simulink model "Questao_5"  (R2023b)
settings: Solver=VariableStepAuto  StartTime=0.0  StopTime=100  RelTol=1e-3
undefined symbols (not defined in the file): B, Kw, Ts
settings Model: Creator=pedro  LastModifiedBy=pedro

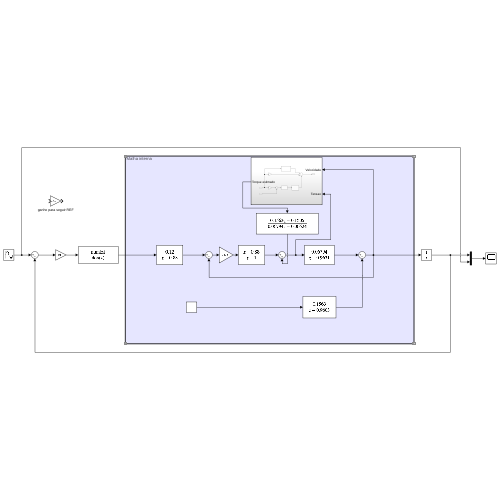
[thumbnail: Simulink's stored preview of the top-level diagram]
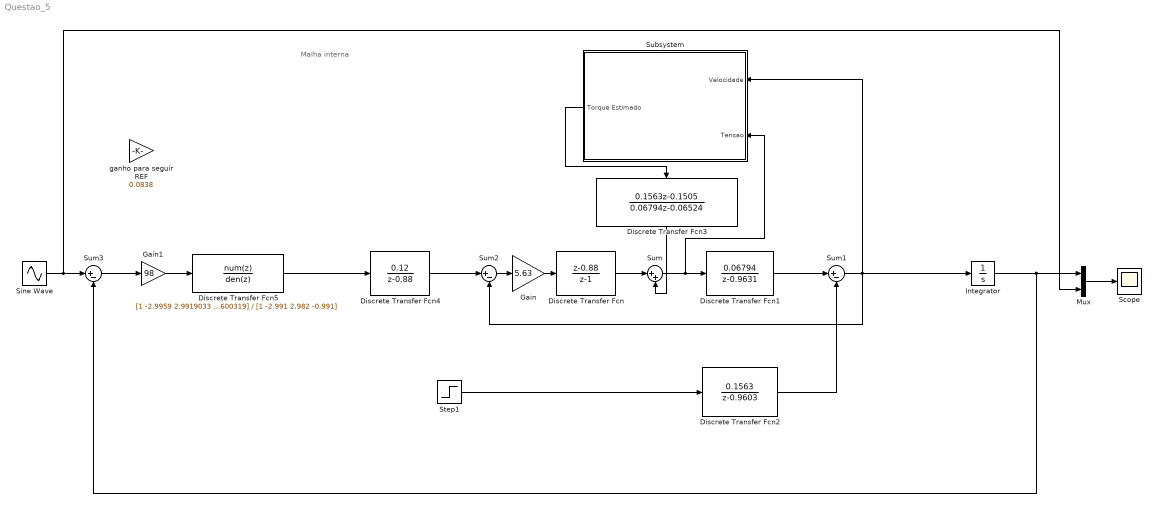
== system Questao_5 ==
  note: Malha interna
  Discrete Transfer Fcn : DiscreteTransferFcn  Numerator=[1 -0.88]  Denominator=[1 -1]
  Discrete Transfer Fcn1 : DiscreteTransferFcn  Numerator=[0.06794]  Denominator=[1 -0.9631]
  Discrete Transfer Fcn2 : DiscreteTransferFcn  Numerator=[0.1563]  Denominator=[1 -0.9603]
  Discrete Transfer Fcn3 : DiscreteTransferFcn  Numerator=[0.1563 -0.1505]  Denominator=[0.06794 -0.06524]
  Discrete Transfer Fcn4 : DiscreteTransferFcn  Numerator=[0.12]  Denominator=[1 -0.88]
  Discrete Transfer Fcn5 : DiscreteTransferFcn  Numerator=[1 -2.9959 2.9919033 -0.99600319]  Denominator=[1 -2.991 2.982 -0.991]
  Gain : Gain  Gain=5.63
  Gain1 : Gain  Gain=98
  Integrator : Integrator
  Mux : Mux  Inputs=2
  Scope : Scope
  Sine Wave : Sin  SampleTime=0.162
  Step1 : Step  Time=10  After=0  SampleTime=0.162
  Subsystem : Subsystem
      settings: PortSchema="{\"entries\":[{\"content\":{\"sides\":[{\"content\":{},\"type\":\"ConnectorPlacement.EquallySpacedRectSide\",\"uuid\":\"e59a06e1-eab4-4bd2-85d9-68e257427de7\"},{\"content\":{\"side\":\"RIGHT\"},\"type\":\"ConnectorPlacement.EquallySpacedRectSide\",\"uuid\":\"6892985a-c8d8-4c3b-9c0c-3e543d6e16eb\"},{\"content\":{\"connectorIds\":[\"Out1\"],\"side\":\"TOP\"},\"type\":\"ConnectorPlacement.EquallySpacedRectSide\",\"uuid\":\"71dba93a-139c-4e39-b2a6-d594bacb8791\"},{\"content\":{\"connectorIds\":[\"In1\",\"In2\"],\"side\":\"BOTTOM\"},\"type\":\"ConnectorPlacement.EquallySpacedRectSide\",\"uuid\":\"1da54c87-6e6c-45c2-97e0-448bf39b9223\"}]},\"type\":\"ConnectorPlacement.EquallySpacedConnector\",\"uuid\":\"3219126c-845c-4a92-9507-56dbcc4fd8de\"}],\"packageUris\":[\"http://schema.mathworks.com/mf0/Connector/R2020b\"],\"version\":\"1.0\"}"
  Sum : Sum  Inputs=|++
  Sum1 : Sum  Inputs=|+-
  Sum2 : Sum  Inputs=|+-
  Sum3 : Sum  Inputs=|+-
  ganho para seguir REF : Gain  Gain=0.0838
  wires:
  Discrete Transfer Fcn/1 -> Sum/1
  Discrete Transfer Fcn4/1 -> Sum2/1
  Discrete Transfer Fcn3/1 -> Sum/2
  Step1/1 -> Discrete Transfer Fcn2/1
  Gain1/1 -> Discrete Transfer Fcn5/1
  Subsystem/1(Torque Estimado) -> Discrete Transfer Fcn3/1
  Sum/1 -> Subsystem/2(Tensao), Discrete Transfer Fcn1/1
  Discrete Transfer Fcn2/1 -> Sum1/2
  Sum2/1 -> Gain/1
  Gain/1 -> Discrete Transfer Fcn/1
  Mux/1 -> Scope/1
  Sum1/1 -> Integrator/1, Subsystem/1(Velocidade), Sum2/2
  Discrete Transfer Fcn1/1 -> Sum1/1
  Integrator/1 -> Mux/1, Sum3/2
  Sum3/1 -> Gain1/1
  Sine Wave/1 -> Mux/2, Sum3/1
  Discrete Transfer Fcn5/1 -> Discrete Transfer Fcn4/1

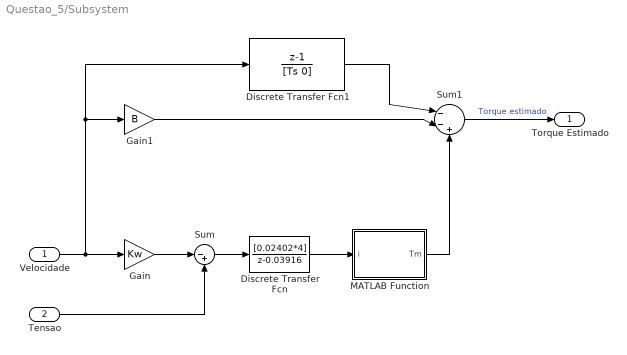
== system Questao_5/Subsystem ==
  Velocidade : Inport
  Tensao : Inport  Port=2
  Discrete Transfer Fcn : DiscreteTransferFcn  Numerator=[0.02402*4]  Denominator=[1 -0.03916]
  Discrete Transfer Fcn1 : DiscreteTransferFcn  Numerator=[1 -1]  Denominator=[Ts 0]
  Gain : Gain  Gain=Kw
  Gain1 : Gain  Gain=B
  MATLAB Function : MATLAB Function  TreatAsAtomicUnit=on
  Sum : Sum  Inputs=|-+
  Sum1 : Sum  Inputs=|--+
  Torque Estimado : Outport
  wires:
  Velocidade/1 -> Discrete Transfer Fcn1/1, Gain1/1, Gain/1
  Gain/1 -> Sum/1
  Tensao/1 -> Sum/2
  Sum/1 -> Discrete Transfer Fcn/1
  Discrete Transfer Fcn/1 -> MATLAB Function/1(i)
  MATLAB Function/1(Tm) -> Sum1/3
  Gain1/1 -> Sum1/2
  Discrete Transfer Fcn1/1 -> Sum1/1
  Sum1/1 -> Torque Estimado/1  "Torque estimado"

== matlab function Questao_5/Subsystem/MATLAB Function ==
  data: i input; Tm output
function Tm = fcn(i)

    if (i < 0)
        Tm = -5.26 * (1 - exp(i));

    else
        Tm = 5.26 * (1 - exp(-i));
    end
